simulink model "M1"  (R2021a)
settings: Solver=VariableStepAuto  StartTime=0.0  StopTime=6  RelTol=1e-3
values from neighbouring files (symbols this model uses):
  A = [-0.127 0 0 0;     0 -0.1512 0 -18.28;     0 1.53 0 288;     0 0 1 0]    [data.m]
  B = [5.77 -5.77;     0.51 0.51;     -5.20 -5.20;     0 0]    [data.m]
  C = [1 0 0 0;     0 1 0 0;     0 0 1 0;     0 0 0 1]    [data.m]
  D = [0 0;     0 0;     0 0;     0 0]    [data.m]    (also in segway.mat = 0.15)
  G_L = G2(1,:)    [data.m]
  G_R = G2(2,:)    [data.m]
  K_L = K2(1,:)    [data.m]
  K_R = K2(2,:)    [data.m]
settings Model: Creator=86198  LastModifiedBy=ivl1
settings SolverCC: AlgebraicLoopSolver=TrustRegion
settings DebuggingCC: SFMachineParentedDataDiag=warning

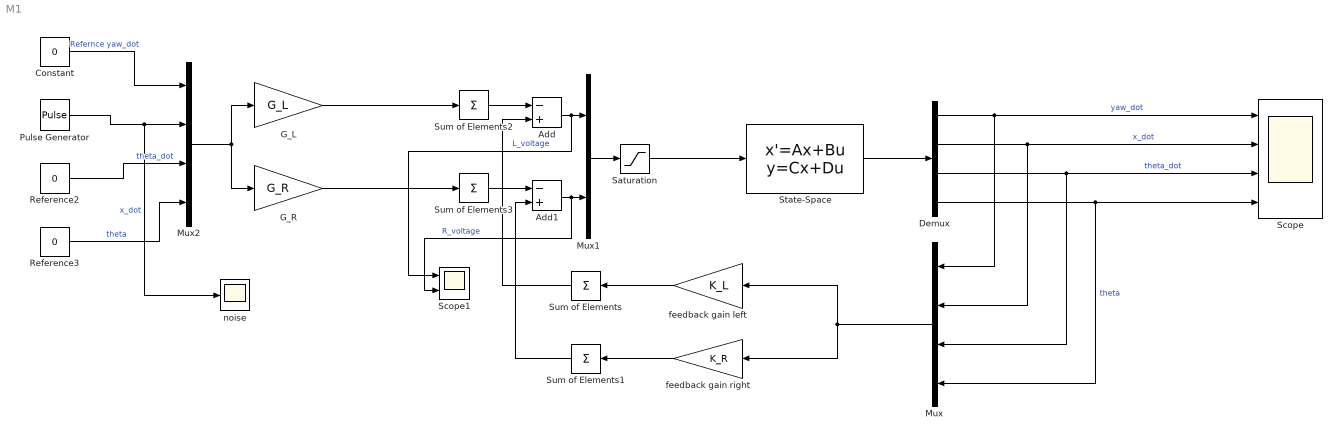
== system M1 ==
  Add : Sum  Inputs=-+
  Add1 : Sum  Inputs=-+
  Constant : Constant  Value=0
  Demux : Demux
  G_L : Gain  Gain=G_L
  G_R : Gain  Gain=G_R
  Mux : Mux
  Mux1 : Mux  Inputs=2
  Mux2 : Mux
  Pulse Generator : DiscretePulseGenerator  PulseType=Time based  Period=10  PhaseDelay=1
  Reference2 : Constant  Value=0
  Reference3 : Constant  Value=0
  Saturation : Saturate  UpperLimit=12  LowerLimit=-12
  Scope : Scope  NumInputPorts=4
  Scope1 : Scope  NumInputPorts=2
  State-Space : StateSpace  A=A  B=B  C=C  D=D  InitialCondition=[0 0 0 0]
  Sum of Elements{,1..3} (4 alike) : Sum  Inputs=+
  feedback gain left : Gain  Gain=K_L
  feedback gain right : Gain  Gain=K_R
  noise : Scope
  wires:
  Mux/1 -> feedback gain right/1, feedback gain left/1
  State-Space/1 -> Demux/1
  Mux1/1 -> Saturation/1
  Add/1 -> Scope1/1, Mux1/1  "L_voltage"
  Add1/1 -> Scope1/2, Mux1/2  "R_voltage"
  feedback gain left/1 -> Sum of Elements/1
  feedback gain right/1 -> Sum of Elements1/1
  Demux/1 -> Scope/1, Mux/1  "yaw_dot"
  Demux/2 -> Scope/2, Mux/2  "x_dot"
  Demux/3 -> Scope/3, Mux/3  "theta_dot"
  Demux/4 -> Scope/4, Mux/4  "theta"
  Sum of Elements/1 -> Add/2
  Sum of Elements1/1 -> Add1/2
  G_L/1 -> Sum of Elements2/1
  G_R/1 -> Sum of Elements3/1
  Sum of Elements2/1 -> Add/1
  Sum of Elements3/1 -> Add1/1
  Saturation/1 -> State-Space/1
  Reference3/1 -> Mux2/4  "theta"
  Constant/1 -> Mux2/1  "Refernce yaw_dot"
  Reference2/1 -> Mux2/3  "theta_dot"
  Pulse Generator/1 -> noise/1, Mux2/2  "x_dot"
  Mux2/1 -> G_R/1, G_L/1
